simulink model "Trial_Merge_Unsuccessful"  (R2020b)
settings: Solver=VariableStepAuto  StartTime=0.0  StopTime=10.0  RelTol=1e-3
values from neighbouring files (symbols this model uses):
  A_2 = zeros(3)    [MPC_tune.m]
  B_2 = I_inv    [MPC_tune.m]
  C_2 = eye(3)    [MPC_tune.m]
  D_2 = zeros(3)    [MPC_tune.m]
  I_inv = inv(I_mat)    [MPC_tune.m]
undefined symbols (not defined in the file or in its folder): Fb1_l, Fb1_u, Fb2_l, Fb2_u, Fb3_l, Fb3_u, Fb4_l, Fb4_u, Fc1_l, Fc1_u, Fc2_l, Fc2_u, Fc3_l, Fc3_u, fprop, Ft1_l, Ft1_u, Ft2_l, Ft2_u, Ft3_l, Ft3_u, Ft4_l, Ft4_u, theta0
libraries: dspsigops x33, pid_lib x3, fuzblock x3, mpclib x1, dspmathops x1
(part 2 of 2)

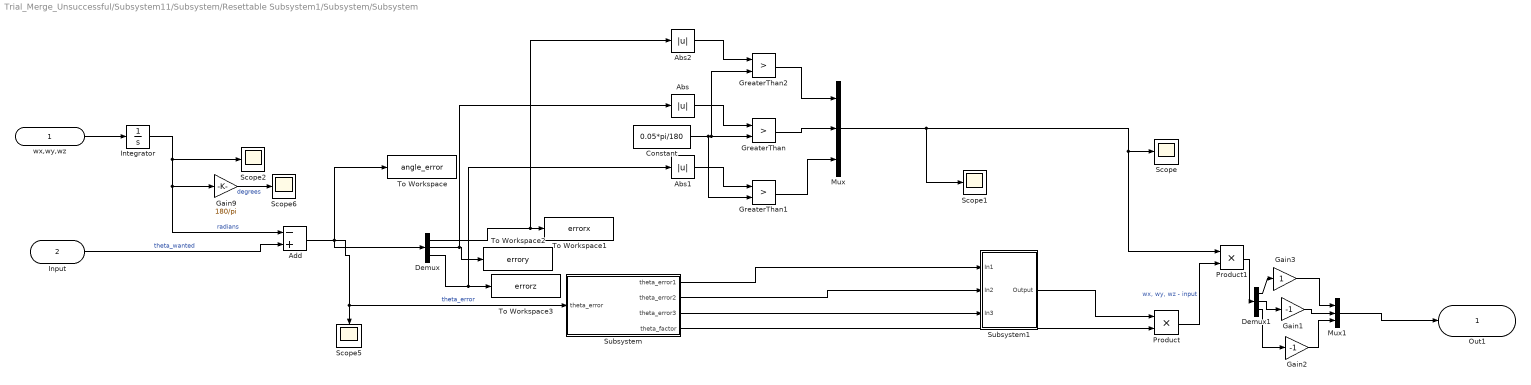
== system Trial_Merge_Unsuccessful/Subsystem11/Subsystem/Resettable Subsystem1/Subsystem/Subsystem ==
  wx,wy,wz : Inport
  Input : Inport  Port=2
  Abs : Abs
  Abs1 : Abs
  Abs2 : Abs
  Add : Sum  Inputs=-+
  Constant : Constant  Value=0.05*pi/180
  Demux : Demux  Outputs=3
  Demux1 : Demux  Outputs=3
  Gain1 : Gain  Gain=-1
  Gain2 : Gain  Gain=-1
  Gain3 : Gain
  Gain9 : Gain  Gain=180/pi
  GreaterThan : RelationalOperator  Operator=>  OutDataTypeStr=boolean  RndMeth=Simplest
  GreaterThan1 : RelationalOperator  Operator=>  OutDataTypeStr=boolean  RndMeth=Simplest
  GreaterThan2 : RelationalOperator  Operator=>  OutDataTypeStr=boolean  RndMeth=Simplest
  Integrator : Integrator  InitialCondition=[0;0;0]
  Mux : Mux  Inputs=3
  Mux1 : Mux  Inputs=3
  Product : Product
  Product1 : Product
  Scope{,1..2,5..6} (5 alike) : Scope
  Subsystem : Subsystem
  Subsystem1 : Subsystem
  To Workspace : ToWorkspace  VariableName=angle_error  SampleTime=-1
  To Workspace1 : ToWorkspace  VariableName=errorx  SaveFormat=Timeseries  SampleTime=-1
      settings: Save2DSignal=2-D array (concatenate along first dimension)
  To Workspace2 : ToWorkspace  VariableName=errory  SaveFormat=Timeseries  SampleTime=-1
  To Workspace3 : ToWorkspace  VariableName=errorz  SaveFormat=Timeseries  SampleTime=-1
  Out1 : Outport
  wires:
  Integrator/1 -> Add/1, Gain9/1, Scope2/1  "radians"
  Add/1 -> To Workspace/1, Demux/1, Subsystem/1(theta_error), Scope5/1  "theta_error"
  Gain9/1 -> Scope6/1  "degrees"
  Input/1 -> Add/2  "theta_wanted"
  Product/1 -> Product1/2  "wx, wy, wz - input"
  wx,wy,wz/1 -> Integrator/1
  Subsystem/4(theta_factor) -> Product/2
  Demux/2 -> Abs/1, To Workspace2/1
  Demux/3 -> Abs1/1, To Workspace3/1
  Demux/1 -> Abs2/1, To Workspace1/1
  Subsystem/1(theta_error1) -> Subsystem1/1(In1)
  Subsystem/2(theta_error2) -> Subsystem1/2(In2)
  Subsystem/3(theta_error3) -> Subsystem1/3(In3)
  Subsystem1/1(Output) -> Product/1
  Abs/1 -> GreaterThan/1
  Constant/1 -> GreaterThan1/2, GreaterThan2/2, GreaterThan/2
  Abs1/1 -> GreaterThan1/1
  Abs2/1 -> GreaterThan2/1
  GreaterThan2/1 -> Mux/1
  GreaterThan/1 -> Mux/2
  GreaterThan1/1 -> Mux/3
  Mux/1 -> Scope1/1, Scope/1, Product1/1
  Product1/1 -> Demux1/1
  Mux1/1 -> Out1/1
  Demux1/2 -> Gain1/1
  Demux1/3 -> Gain2/1
  Demux1/1 -> Gain3/1
  Gain3/1 -> Mux1/1
  Gain1/1 -> Mux1/2
  Gain2/1 -> Mux1/3

== system Trial_Merge_Unsuccessful/Subsystem11/Subsystem/Resettable Subsystem1/Subsystem/Subsystem1 ==
  u : Inport
  A : Inport  Port=2
  B : Inport  Port=3
  C : Inport  Port=4
  D : Inport  Port=5
  w_0 : Inport  Port=6
  Input : Inport  Port=7
  Product{,1..3} (4 alike) : Product  SCDEnableBlockLinearizationSpecification=on  Multiplication=Matrix(*)
  Resettable Subsystem : Subsystem  TreatAsAtomicUnit=on
  Sum : Sum  Inputs=|++
  Sum1 : Sum  Inputs=++|
  dxTerm : Terminator
  y : Outport  VectorParamsAs1DForOutWhenUnconnected=off
  x : Outport  Port=2  VectorParamsAs1DForOutWhenUnconnected=off
  wires:
  Sum/1 -> Resettable Subsystem/1(alpha), dxTerm/1  "dx"
  Product3/1 -> Sum1/1  "Cx"
  Product/1 -> Sum/1  "Bu"
  u/1 -> Product2/2, Product/2
  Product2/1 -> Sum1/2  "Du"
  Resettable Subsystem/1(x) -> x/1, Product1/2, Product3/2  "x"
  A/1 -> Product1/1
  Product1/1 -> Sum/2  "Ax"
  C/1 -> Product3/1
  B/1 -> Product/1
  D/1 -> Product2/1
  Sum1/1 -> y/1
  w_0/1 -> Resettable Subsystem/2(omega0)
  Input/1 -> Resettable Subsystem/Reset

== system Trial_Merge_Unsuccessful/Subsystem11/Subsystem/Resettable Subsystem1/Subsystem1/Subsystem ==
  F_c_d : Inport
  M_c_d : Inport  Port=2
  Demux8 : Demux  Outputs=3
  Demux9 : Demux  Outputs=3
  MATLAB Function : MATLAB Function  TreatAsAtomicUnit=on
  MATLAB Function6 : MATLAB Function  TreatAsAtomicUnit=on
  Mux23 : Mux
  Mux24 : Mux
  Mux9 : Mux  Inputs=3
  Terminator12 : Terminator
  To Workspace6 : ToWorkspace  VariableName=Fc_wanted  SaveFormat=Timeseries  SampleTime=-1
  To Workspace7 : ToWorkspace  VariableName=Ft_wanted  SaveFormat=Timeseries  SampleTime=-1
  To Workspace8 : ToWorkspace  VariableName=Fb_wanted  SaveFormat=Timeseries  SampleTime=-1
  Fb_wanted : Outport
  Ft_wanted : Outport  Port=2
  Fc_wanted : Outport  Port=3
  wires:
  Demux9/3 -> MATLAB Function6/3(M_z)
  Demux8/2 -> MATLAB Function6/1(F_y)
  Mux9/1 -> Fc_wanted/1, To Workspace6/1  "Fc_wanted"
  MATLAB Function/2(Ft2) -> Mux23/2  "Fb_wanted"
  Demux9/1 -> MATLAB Function6/2(M_x)
  MATLAB Function/3(Ft3) -> Mux23/3
  Demux9/2 -> MATLAB Function/1(My)
  MATLAB Function/8(Fb4) -> Mux24/4
  MATLAB Function6/1(F_c1) -> Mux9/1
  MATLAB Function/1(Ft1) -> Mux23/1  "Ft_wanted"
  Demux8/1 -> Terminator12/1
  Mux23/1 -> Ft_wanted/1, To Workspace7/1  "Ft_wanted"
  Mux24/1 -> Fb_wanted/1, To Workspace8/1  "Fb_wanted"
  MATLAB Function6/3(F_c3) -> Mux9/3
  MATLAB Function/5(Fb1) -> Mux24/1
  MATLAB Function/6(Fb2) -> Mux24/2
  MATLAB Function/7(Fb3) -> Mux24/3
  MATLAB Function/4(Ft4) -> Mux23/4
  Demux8/3 -> MATLAB Function/2(Fz)
  MATLAB Function6/2(F_c2) -> Mux9/2
  F_c_d/1 -> Demux8/1
  M_c_d/1 -> Demux9/1

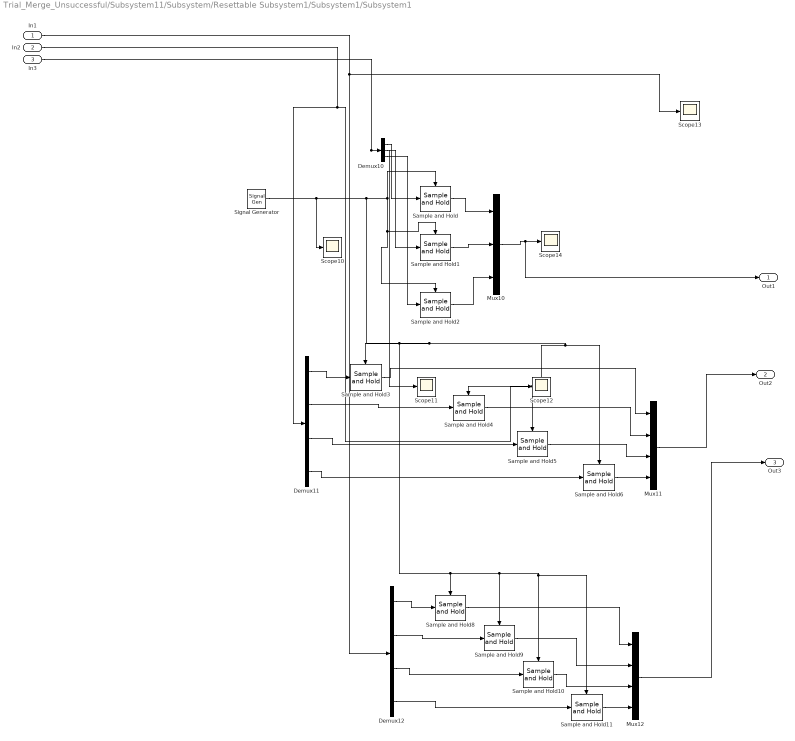
== system Trial_Merge_Unsuccessful/Subsystem11/Subsystem/Resettable Subsystem1/Subsystem1/Subsystem1 ==
  In1 : Inport
  In2 : Inport  Port=2
  In3 : Inport  Port=3
  Demux10 : Demux  Outputs=3
  Demux11 : Demux
  Demux12 : Demux
  Mux10 : Mux  Inputs=3
  Mux11 : Mux
  Mux12 : Mux
  Sample and Hold{,1..6,8..11} (11 alike) : dspsigops/Sample and Hold  trig=Rising edge  initCond=0  latchinput=off
  Scope{10..14} (5 alike) : Scope
  Signal Generator : SignalGenerator  WaveForm=square  Frequency=fprop  Units=rad/sec
  Out1 : Outport
  Out2 : Outport  Port=2
  Out3 : Outport  Port=3
  wires:
  Demux12/1 -> Sample and Hold8/1
  Demux11/1 -> Sample and Hold3/1
  Signal Generator/1 -> Scope10/1, Sample and Hold11/Trigger, Sample and Hold10/Trigger, Sample and Hold9/Trigger, Sample and Hold8/Trigger, Sample and Hold4/Trigger, Sample and Hold5/Trigger, Sample and Hold6/Trigger, Sample and Hold3/Trigger, Sample and Hold/Trigger, Sample and Hold2/Trigger, Sample and Hold1/Trigger
  In2/1 -> Scope12/1, Demux11/1
  In3/1 -> Scope11/1, Demux10/1
  Demux10/3 -> Sample and Hold2/1
  Sample and Hold10/1 -> Mux12/3
  Sample and Hold/1 -> Mux10/1
  Demux12/4 -> Sample and Hold11/1
  Sample and Hold6/1 -> Mux11/4
  Demux10/1 -> Sample and Hold/1
  Mux10/1 -> Out1/1, Scope14/1
  Demux12/3 -> Sample and Hold10/1
  Sample and Hold8/1 -> Mux12/1
  Sample and Hold3/1 -> Mux11/1
  Sample and Hold5/1 -> Mux11/3
  Sample and Hold1/1 -> Mux10/2
  Sample and Hold11/1 -> Mux12/4
  In1/1 -> Scope13/1, Demux12/1
  Demux10/2 -> Sample and Hold1/1
  Demux11/2 -> Sample and Hold4/1
  Sample and Hold2/1 -> Mux10/3
  Sample and Hold4/1 -> Mux11/2
  Sample and Hold9/1 -> Mux12/2
  Demux11/3 -> Sample and Hold5/1
  Mux12/1 -> Out3/1
  Demux12/2 -> Sample and Hold9/1
  Demux11/4 -> Sample and Hold6/1
  Mux11/1 -> Out2/1

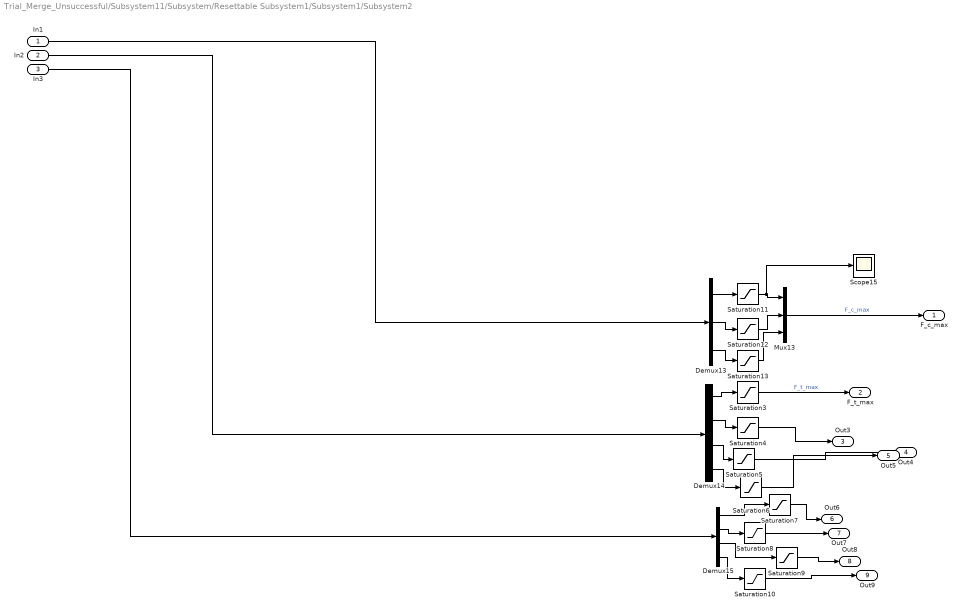
== system Trial_Merge_Unsuccessful/Subsystem11/Subsystem/Resettable Subsystem1/Subsystem1/Subsystem2 ==
  In1 : Inport
  In2 : Inport  Port=2
  In3 : Inport  Port=3
  Demux13 : Demux  Outputs=3
  Demux14 : Demux
  Demux15 : Demux
  Mux13 : Mux  Inputs=3
  Saturation10 : Saturate  UpperLimit=Fb4_u  LowerLimit=Fb4_l
  Saturation11 : Saturate  UpperLimit=Fc1_u  LowerLimit=Fc1_l
  Saturation12 : Saturate  UpperLimit=Fc2_u  LowerLimit=Fc2_l
  Saturation13 : Saturate  UpperLimit=Fc3_u  LowerLimit=Fc3_l
  Saturation3 : Saturate  UpperLimit=Ft1_u  LowerLimit=Ft1_l
  Saturation4 : Saturate  UpperLimit=Ft2_u  LowerLimit=Ft2_l
  Saturation5 : Saturate  UpperLimit=Ft3_u  LowerLimit=Ft3_l
  Saturation6 : Saturate  UpperLimit=Ft4_u  LowerLimit=Ft4_l
  Saturation7 : Saturate  UpperLimit=Fb1_u  LowerLimit=Fb1_l
  Saturation8 : Saturate  UpperLimit=Fb2_u  LowerLimit=Fb2_l
  Saturation9 : Saturate  UpperLimit=Fb3_u  LowerLimit=Fb3_l
  Scope15 : Scope
  F_c_max : Outport
  F_t_max : Outport  Port=2
  Out3 : Outport  Port=3
  Out4 : Outport  Port=4
  Out5 : Outport  Port=5
  Out6 : Outport  Port=6
  Out7 : Outport  Port=7
  Out8 : Outport  Port=8
  Out9 : Outport  Port=9
  wires:
  Saturation11/1 -> Scope15/1, Mux13/1
  Demux13/2 -> Saturation12/1
  Saturation10/1 -> Out9/1
  Demux13/3 -> Saturation13/1
  Demux14/1 -> Saturation3/1
  Demux14/4 -> Saturation6/1
  In3/1 -> Demux15/1
  Demux14/3 -> Saturation5/1
  Demux13/1 -> Saturation11/1
  Saturation13/1 -> Mux13/3
  In1/1 -> Demux13/1
  Demux15/1 -> Saturation7/1
  Demux15/2 -> Saturation8/1
  Demux15/3 -> Saturation9/1
  Saturation12/1 -> Mux13/2
  Demux15/4 -> Saturation10/1
  Demux14/2 -> Saturation4/1
  Saturation9/1 -> Out8/1
  Saturation5/1 -> Out4/1
  In2/1 -> Demux14/1
  Saturation4/1 -> Out3/1
  Saturation7/1 -> Out6/1
  Mux13/1 -> F_c_max/1  "F_c_max"
  Saturation6/1 -> Out5/1
  Saturation3/1 -> F_t_max/1  "F_t_max"
  Saturation8/1 -> Out7/1

== system Trial_Merge_Unsuccessful/Subsystem11/Subsystem/Resettable Subsystem1/Subsystem1/Subsystem3 ==
  In1 : Inport
  In2 : Inport  Port=2
  In3 : Inport  Port=3
  Ft3 : Inport  Port=4
  Ft4 : Inport  Port=5
  Fb1 : Inport  Port=6
  In7 : Inport  Port=7
  Fb3 : Inport  Port=8
  In9 : Inport  Port=9
  Constant23 : Constant  Value=0
  Demux16 : Demux  Outputs=3
  MATLAB Function7 : MATLAB Function  TreatAsAtomicUnit=on
  MATLAB Function8 : MATLAB Function  TreatAsAtomicUnit=on
  MATLAB Function9 : MATLAB Function  TreatAsAtomicUnit=on
  Mux : Mux
  Mux1 : Mux
  Mux16 : Mux  Inputs=3
  Mux17 : Mux  Inputs=3
  To Workspace : ToWorkspace  VariableName=Fc  SaveFormat=Timeseries  SampleTime=-1
  To Workspace1 : ToWorkspace  VariableName=Ft  SaveFormat=Timeseries  SampleTime=-1
  To Workspace2 : ToWorkspace  VariableName=Fb  SaveFormat=Timeseries  SampleTime=-1
  Out1 : Outport
  Mc(t-tau)_actual : Outport  Port=2
  wires:
  Demux16/2 -> MATLAB Function8/2(F_c2)
  In9/1 -> Mux1/4, MATLAB Function9/8(Fb4)
  In3/1 -> Mux/2, MATLAB Function9/2(Ft2)
  MATLAB Function7/1(F_z) -> Mux16/3  "Fz_actual"
  In1/1 -> Demux16/1, To Workspace/1
  Fb3/1 -> Mux1/3, MATLAB Function9/7(Fb3)
  MATLAB Function9/1(F1) -> MATLAB Function7/1(F1)
  Ft3/1 -> Mux/3, MATLAB Function9/3(Ft3)
  MATLAB Function8/1(F_y) -> Mux16/2  "Fy_actual"
  Fb1/1 -> Mux1/1, MATLAB Function9/5(Fb1)
  MATLAB Function8/3(M_z) -> Mux17/3  "M_z_acc"
  MATLAB Function7/2(M_y) -> Mux17/2  "M_y_acc"
  Mux17/1 -> Mc(t-tau)_actual/1  "Mc(t-tau)_actual"
  Ft4/1 -> Mux/4, MATLAB Function9/4(Ft4)
  MATLAB Function8/2(M_x) -> Mux17/1  "M_x_acc"
  In7/1 -> Mux1/2, MATLAB Function9/6(Fb2)
  MATLAB Function9/3(F3) -> MATLAB Function7/3(F3)
  Demux16/1 -> MATLAB Function8/1(F_c1)
  Constant23/1 -> Mux16/1  "Fx_actual"
  In2/1 -> Mux/1, MATLAB Function9/1(Ft1)
  MATLAB Function9/2(F2) -> MATLAB Function7/2(F2)
  Mux1/1 -> To Workspace2/1
  Demux16/3 -> MATLAB Function8/3(F_c3)
  Mux/1 -> To Workspace1/1
  Mux16/1 -> Out1/1

== system Trial_Merge_Unsuccessful/Subsystem11/Subsystem/Resettable Subsystem1/Subsystem1/Subsystem4 ==
  TVd : Inport
  In2 : Inport  Port=2
  Constant24 : Constant  Value=[0;1;1]
  Matrix Multiply3 : Product  Multiplication=Matrix(*)
  Product5 : Product
  Fc(t-tau)_actual : Outport
  Fc(t-tau)_actual1 : Outport  Port=2
  wires:
  Matrix Multiply3/1 -> Fc(t-tau)_actual1/1, Product5/2  "Fc(t-tau)_actual"
  Constant24/1 -> Product5/1
  TVd/1 -> Matrix Multiply3/1
  Product5/1 -> Fc(t-tau)_actual/1  "Fc(t-tau)_actual"
  In2/1 -> Matrix Multiply3/2

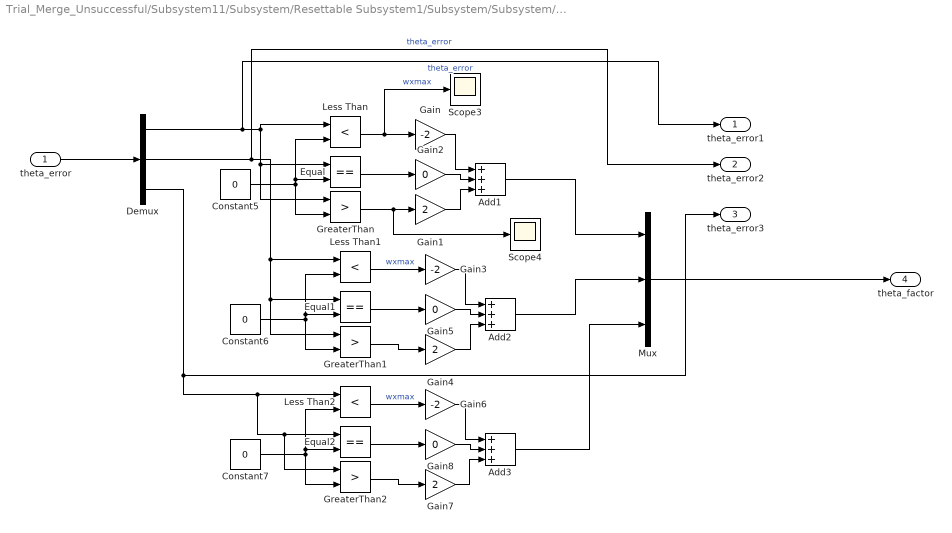
== system Trial_Merge_Unsuccessful/Subsystem11/Subsystem/Resettable Subsystem1/Subsystem/Subsystem/Subsystem ==
  theta_error : Inport
  Add1 : Sum  Inputs=+++
  Add2 : Sum  Inputs=+++
  Add3 : Sum  Inputs=+++
  Constant5 : Constant  Value=0
  Constant6 : Constant  Value=0
  Constant7 : Constant  Value=0
  Demux : Demux  Outputs=3
  Equal : RelationalOperator  Operator===  OutDataTypeStr=boolean  RndMeth=Simplest
  Equal1 : RelationalOperator  Operator===  OutDataTypeStr=boolean  RndMeth=Simplest
  Equal2 : RelationalOperator  Operator===  OutDataTypeStr=boolean  RndMeth=Simplest
  Gain : Gain  Gain=-2
  Gain1 : Gain  Gain=2
  Gain2 : Gain  Gain=0
  Gain3 : Gain  Gain=-2
  Gain4 : Gain  Gain=2
  Gain5 : Gain  Gain=0
  Gain6 : Gain  Gain=-2
  Gain7 : Gain  Gain=2
  Gain8 : Gain  Gain=0
  GreaterThan : RelationalOperator  Operator=>  OutDataTypeStr=boolean  RndMeth=Simplest
  GreaterThan1 : RelationalOperator  Operator=>  OutDataTypeStr=boolean  RndMeth=Simplest
  GreaterThan2 : RelationalOperator  Operator=>  OutDataTypeStr=boolean  RndMeth=Simplest
  Less Than : RelationalOperator  Operator=<  OutDataTypeStr=boolean  RndMeth=Simplest
  Less Than1 : RelationalOperator  Operator=<  OutDataTypeStr=boolean  RndMeth=Simplest
  Less Than2 : RelationalOperator  Operator=<  OutDataTypeStr=boolean  RndMeth=Simplest
  Mux : Mux  Inputs=3
  Scope3 : Scope
  Scope4 : Scope
  theta_error1 : Outport
  theta_error2 : Outport  Port=2
  theta_error3 : Outport  Port=3
  theta_factor : Outport  Port=4
  wires:
  Add1/1 -> Mux/1
  Constant5/1 -> Equal/2, Less Than/2, GreaterThan/2
  Equal2/1 -> Gain8/1
  Demux/1 -> theta_error1/1, GreaterThan/1, Equal/1, Less Than/1  "theta_error"
  GreaterThan2/1 -> Gain7/1
  Gain1/1 -> Add1/3
  Gain7/1 -> Add3/3
  Less Than1/1 -> Gain3/1  "wxmax"
  Gain6/1 -> Add3/1
  Equal/1 -> Gain2/1
  Gain5/1 -> Add2/2
  Add3/1 -> Mux/3
  GreaterThan/1 -> Scope4/1, Gain1/1
  Constant6/1 -> Equal1/2, Less Than1/2, GreaterThan1/2
  Demux/3 -> theta_error3/1, GreaterThan2/1, Equal2/1, Less Than2/1
  Gain3/1 -> Add2/1
  Constant7/1 -> Equal2/2, Less Than2/2, GreaterThan2/2
  Equal1/1 -> Gain5/1
  Gain8/1 -> Add3/2
  Gain4/1 -> Add2/3
  GreaterThan1/1 -> Gain4/1
  Gain/1 -> Add1/1
  Demux/2 -> theta_error2/1, GreaterThan1/1, Equal1/1, Less Than1/1  "theta_error"
  Gain2/1 -> Add1/2
  Add2/1 -> Mux/2
  Less Than/1 -> Scope3/1, Gain/1  "wxmax"
  Less Than2/1 -> Gain6/1  "wxmax"
  theta_error/1 -> Demux/1
  Mux/1 -> theta_factor/1

== system Trial_Merge_Unsuccessful/Subsystem11/Subsystem/Resettable Subsystem1/Subsystem/Subsystem/Subsystem1 ==
  In1 : Inport
  In2 : Inport  Port=2
  In3 : Inport  Port=3
  Abs : Abs
  Abs1 : Abs
  Abs2 : Abs
  Demux : Demux  Outputs=3
  Gain : Gain  Gain=10
  Gain1 : Gain  Gain=125
  Gain10 : Gain  Gain=125
  Gain2 : Gain  Gain=125
  Gain3 : Gain  Gain=10
  Gain4 : Gain  Gain=10
  Mux : Mux  Inputs=3
  Mux1 : Mux  Inputs=3
  Normalization : dspmathops/Normalization  NormType=Squared 2-norm  Bias=1e-10  NormOver=Each column  Dimension=1  roundingMode=Floor  overflowMode=off  accumDataTypeStr=Inherit: Same as product output  accumLastDataTypeStr=Inherit: Same as product output  outputDataTypeStr=Inherit: Same as product output  outputMin=[]  outputMax=[]  outputLastDataTypeStr=Inherit: Same as product output
  Scope{,1..7} (8 alike) : Scope
  Sigmoidal MF : fuzblock/Membership  Functions/Sigmoidal MF  a=10^(-8)  c=1000
      settings: SourceProductBaseCode=FL
  Sigmoidal MF1 : fuzblock/Membership  Functions/Sigmoidal MF  a=10^(-8)  c=1000
      settings: SourceProductBaseCode=FL
  Sigmoidal MF2 : fuzblock/Membership  Functions/Sigmoidal MF  a=10^(-8)  c=1000
      settings: SourceProductBaseCode=FL
  Output : Outport
  wires:
  Gain2/1 -> Mux/2
  Gain10/1 -> Mux/1
  Sigmoidal MF1/1 -> Gain1/1, Scope1/1
  Sigmoidal MF/1 -> Gain10/1, Scope7/1
  Sigmoidal MF2/1 -> Gain2/1, Scope3/1
  Gain/1 -> Scope/1, Sigmoidal MF/1
  Gain1/1 -> Mux/3
  Gain3/1 -> Scope2/1, Sigmoidal MF2/1
  In2/1 -> Abs1/1
  In1/1 -> Abs/1
  In3/1 -> Abs2/1
  Mux/1 -> Output/1
  Abs/1 -> Mux1/1
  Abs1/1 -> Mux1/2
  Gain4/1 -> Scope4/1, Sigmoidal MF1/1
  Abs2/1 -> Mux1/3
  Demux/3 -> Gain4/1
  Demux/1 -> Gain/1
  Demux/2 -> Gain3/1
  Mux1/1 -> Normalization/1, Scope6/1
  Normalization/1 -> Scope5/1, Demux/1

== system Trial_Merge_Unsuccessful/Subsystem11/Subsystem/Resettable Subsystem1/Subsystem/Subsystem1/Resettable Subsystem ==
  alpha : Inport
  omega0 : Inport  Port=2
  Reset : ResetPort  DisableCoverage=on
  Integrator : Integrator  InitialConditionSource=external  InitialCondition=theta0
  Scope : Scope
  x : Outport
  wires:
  omega0/1 -> Integrator/2
  alpha/1 -> Integrator/1
  Integrator/1 -> Scope/1, x/1

== matlab function Trial_Merge_Unsuccessful/Subsystem11/Subsystem/Resettable Subsystem/Subsystem/Subsystem3/MATLAB Function9 ==
  data: Ft1 input; F1 output; Ft2 input; F2 output; F3 output; Ft3 input; Ft4 input; Fb1 input; Fb2 input; Fb3 input; Fb4 input
function [F1, F2, F3] = fcn(Ft1, Ft2, Ft3, Ft4, Fb1, Fb2, Fb3, Fb4)
%F3 is one prop
%F1 is two props
%F2 is two props
F1 = 2*Ft1;
F2 = 2*Fb1;
F3 = Ft3;
end

== matlab function Trial_Merge_Unsuccessful/Subsystem5/MATLAB Function5 ==
  data: M_y input; F1 output; F_z input; F2 output; F3 output
function [F1, F2, F3] = fcn(M_y, F_z)
xt_1 = 1.2598;
xb_1 = 2.2598;
xt_3 = -1.3402;
x_t1 = xt_1;
x_b1 = xb_1;
x_t3 = xt_3;



A_mat = [1 1;
    xt_1 xb_1];

A_inv = inv(A_mat);

p_0 = 0.2;
p_minus1 = 0;
step = 1000;
Converged = 0;
p_list = [];
x_list = [];
y_list = [];
J_list = [];
Fzz =[];
Myy =[];
while Converged == 0
    B = [(F_z - 4*p_0); (M_y - 4*p_0*xt_3)];
    force_0 = (A_inv*B);
    J_0 = sqrt(force_0(1)^2 + force_0(2)^2 + p_0^2);
    back = A_mat*force_0;
    backtrack = [4*p_0; 4*p_0*xt_3];
    forceback = back+backtrack;
    diff = sum(abs(forceback - [F_z; M_y]));
    if diff > 10^(-7)
        disp('Error')
        break
    end
    force = force_0;
    J = J_0;
    p = p_0;
    
    p_1 = p_0 + step;
    B = [(F_z - 4*p_1); (M_y - 4*p_1*xt_3)];
    force_1 = (A_inv*B);
    J_1 = sqrt(force_1(1)^2 + force_1(2)^2 + p_1^2);
    back = A_mat*force_1;
    backtrack = [4*p_1; 4*p_1*xt_3];
    forceback = back+backtrack;
    diff = sum(abs(forceback - [F_z; M_y]));
    if diff > 10^(-7)
        disp('Error')
        break
    end
    if J_1 < J_0
        force = force_1;
        J = J_1;
        p = p_1;
    end
    
    p_2 = p_0 - step;
    B = [(F_z - 4*p_2); (M_y - 4*p_2*xt_3)];
    force_2 = (A_inv*B);
    J_2 = sqrt(force_2(1)^2 + force_2(2)^2 + p_2^2);
    back = A_mat*force_2;
    backtrack = [4*p_2; 4*p_2*xt_3];
    forceback = back+backtrack;
    diff = sum(abs(forceback - [F_z; M_y]));
    if diff > 10^(-7)
        disp('Error')
        break
    end
    if J_2 < J_0 && J_2 < J_1
        force = force_2;
        J = J_2;
        p = p_2;
    end
    
    if p_minus1 < p_0 && p_0 < p
        step = step;
    elseif p_minus1 > p_0 && p_0 > p
        step = step;
    else
        step = step*0.9;
    end
        
    p_minus1 = p_0;
    p_0 = p;
    p_list = [p_list; p_0];
    x_list = [x_list; force(1)];
    y_list = [y_list; force(2)];
    J_list = [J_list; J];
    if step < abs(min([F_z,M_y])*10^(-9))
        Converged = 1;
    end
    
    
end

F1 = x_list(length(x_list));
F2 = y_list(length(y_list));
F3 = p_0;
end

== matlab function Trial_Merge_Unsuccessful/Subsystem5/Subsystem/MATLAB Function6 ==
  data: F_y input; F_c1 output; M_x input; M_z input; F_c2 output; F_c3 output
function [F_c1, F_c2, F_c3] = fcn(F_y, M_x, M_z)
%CATIA trans
TcgCatia = [1 0 0;
    0 -1 0;
    0 0 -1];

%Propeller arms - changed due to CATIA errors
c_1 = [-640.1998; 0; 506.566]*10^(-3);      %Control Back Top
c_2 = [-1040.1998; 0; -493.434]*10^(-3);    %Control Back Bottom
c_3 = [2259.8002; 0; -293.434]*10^(-3);     %Control Front

%Propeller arms - rotated
c_1 = TcgCatia*c_1;
c1 = transpose(c_1);
c_2 = TcgCatia*c_2;
c2 = transpose(c_2);
c_3 = TcgCatia*c_3;
c3 = transpose(c_3);

xc_1 = c1(1);
zc_1 = c1(3);

xc_2 = c2(1);
zc_2 = c2(3);

xc_3 = c3(1);
zc_3 = c3(3);

A_control = [1 1 1;
    zc_1 zc_2 zc_3;
    xc_1 xc_2 xc_3];
A_cinv = inv(A_control);
force_control = [F_y; M_x; M_z];
controlvec = A_cinv*force_control;
F_c1 = controlvec(1);
F_c2 = controlvec(2);
F_c3 = controlvec(3);
end

== matlab function Trial_Merge_Unsuccessful/Subsystem5/MATLAB Function4 ==
  data: F1 input; F_t1 output; F2 input; F3 input; F_t2 output; F_t3 output; F_t4 output; F_b1 output; F_b2 output; F_b3 output; F_b4 output
function [F_t1, F_t2, F_t3, F_t4, F_b1, F_b2, F_b3, F_b4] = fcn(F1, F2, F3)
%F3 is one prop
%F1 is two props
%F2 is two props
F_t1 = F1/2;
F_t2 = F_t1;
F_t3 = F3;
F_t4 = F_t3;
F_b3 = F_t3;
F_b4 = F_t3;
F_b1 = F2/2;
F_b2 = F_b1;

Ft = [F_t1, F_t2, F_t3, F_t4];
Fb = [F_b1, F_b2, F_b3, F_b4];
end

== matlab function Trial_Merge_Unsuccessful/Subsystem5/Subsystem3/MATLAB Function7 ==
  data: F1 input; F_z output; F2 input; M_y output; F3 input
function [F_z, M_y] = fcn(F1, F2, F3)
xt_1 = 1.2598;
xb_1 = 2.2598;
xt_3 = -1.3402;
x_t1 = xt_1;
x_b1 = xb_1;
x_t3 = xt_3;

M_y = -100;
F_z = 0;

A_mat = [1 1;
    xt_1 xb_1];

A_inv = inv(A_mat);

force = [F1; F2];

back = A_mat*force;
backtrack = [4*F3; 4*F3*xt_3];
forceback = back+backtrack;
F_z = forceback(1);
M_y = forceback(2) + 0.15;
end

== matlab function Trial_Merge_Unsuccessful/Subsystem5/Subsystem3/MATLAB Function8 ==
  data: F_c1 input; F_y output; M_x output; F_c2 input; F_c3 input; M_z output
function [F_y, M_x, M_z] = fcn(F_c1, F_c2, F_c3)

%CATIA trans
TcgCatia = [1 0 0;
    0 -1 0;
    0 0 -1];

%Propeller arms - changed due to CATIA errors
c_1 = [-640.1998; 0; 506.566]*10^(-3);      %Control Back Top
c_2 = [-1040.1998; 0; -493.434]*10^(-3);    %Control Back Bottom
c_3 = [2259.8002; 0; -293.434]*10^(-3);     %Control Front

%Propeller arms - rotated
c_1 = TcgCatia*c_1;
c1 = transpose(c_1);
c_2 = TcgCatia*c_2;
c2 = transpose(c_2);
c_3 = TcgCatia*c_3;
c3 = transpose(c_3);

xc_1 = c1(1);
zc_1 = c1(3);

xc_2 = c2(1);
zc_2 = c2(3);

xc_3 = c3(1);
zc_3 = c3(3);


Control_forces = [F_c1; F_c2; F_c3];

A_control = [1 1 1;
        zc_1 zc_2 zc_3;
        xc_1 xc_2 xc_3]; 
Control_vec_2 = A_control*Control_forces;
F_y = Control_vec_2(1);
M_x = Control_vec_2(2);
M_z = Control_vec_2(3);
end

== matlab function Trial_Merge_Unsuccessful/Subsystem5/Subsystem3/MATLAB Function9 ==
  data: Ft1 input; F1 output; Ft2 input; F2 output; F3 output; Ft3 input; Ft4 input; Fb1 input; Fb2 input; Fb3 input; Fb4 input
function [F1, F2, F3] = fcn(Ft1, Ft2, Ft3, Ft4, Fb1, Fb2, Fb3, Fb4)
%F3 is one prop
%F1 is two props
%F2 is two props
F1 = 2*Ft1;
F2 = 2*Fb1;
F3 = Ft3;
end

== matlab function Trial_Merge_Unsuccessful/Subsystem11/Subsystem/Resettable Subsystem/Subsystem/MATLAB Function4 ==
  data: F1 input; F_t1 output; F2 input; F3 input; F_t2 output; F_t3 output; F_t4 output; F_b1 output; F_b2 output; F_b3 output; F_b4 output
function [F_t1, F_t2, F_t3, F_t4, F_b1, F_b2, F_b3, F_b4] = fcn(F1, F2, F3)
%F3 is one prop
%F1 is two props
%F2 is two props
F_t1 = F1/2;
F_t2 = F_t1;
F_t3 = F3;
F_t4 = F_t3;
F_b3 = F_t3;
F_b4 = F_t3;
F_b1 = F2/2;
F_b2 = F_b1;

Ft = [F_t1, F_t2, F_t3, F_t4];
Fb = [F_b1, F_b2, F_b3, F_b4];
end

== matlab function Trial_Merge_Unsuccessful/Subsystem11/Subsystem/Resettable Subsystem/Subsystem4/MATLAB Function2 ==
  data: theta_x input; Transformation_Mat output; theta_y input; theta_z input
function Transformation_Mat  = Euler(theta_x, theta_y, theta_z)

a = cos(theta_x)*cos(theta_z);
b = cos(theta_x)*sin(theta_z);
c = - sin(theta_x);
d = sin(theta_y)*sin(theta_x)*cos(theta_z) - cos(theta_y)*sin(theta_z);
e = sin(theta_y)*sin(theta_x)*sin(theta_z) + cos(theta_y)*cos(theta_z);
f = sin(theta_y)*cos(theta_x);
g = cos(theta_y)*sin(theta_x)*cos(theta_z) + sin(theta_y)*sin(theta_z);
h = cos(theta_y)*sin(theta_x)*sin(theta_z) - sin(theta_y)*cos(theta_z);
i = cos(theta_y)*cos(theta_x);

Transformation_Mat = [a b c;
    d e f;
    g h i];


end

== matlab function Trial_Merge_Unsuccessful/Subsystem11/Subsystem/Resettable Subsystem/Subsystem4/MATLAB Function3 ==
  data: theta_x input; Transformation_Mat output; theta_y input; theta_z input
function Transformation_Mat  = Euler(theta_x, theta_y, theta_z)

a = cos(theta_x)*cos(theta_z);
b = cos(theta_x)*sin(theta_z);
c = - sin(theta_x);
d = sin(theta_y)*sin(theta_x)*cos(theta_z) - cos(theta_y)*sin(theta_z);
e = sin(theta_y)*sin(theta_x)*sin(theta_z) + cos(theta_y)*cos(theta_z);
f = sin(theta_y)*cos(theta_x);
g = cos(theta_y)*sin(theta_x)*cos(theta_z) + sin(theta_y)*sin(theta_z);
h = cos(theta_y)*sin(theta_x)*sin(theta_z) - sin(theta_y)*cos(theta_z);
i = cos(theta_y)*cos(theta_x);

Transformation_Mat = [a b c;
    d e f;
    g h i];


end

== matlab function Trial_Merge_Unsuccessful/Subsystem11/Subsystem/Resettable Subsystem/Subsystem3/MATLAB Function10 ==
  settings: updateMethod=DISCRETE
  data: xvel input; yvel input; zvel input; wx output; accx input; accy input; accz input; wy output; wz output
function [wx, wy, wz]  = fungyroscope(xvel, yvel, zvel, accx, accy, accz)
   
    % Create gyroscope sensor object
    params = gyroparams;         
    
    % Parameters for simulated signal
    N = 1;       % Number of samples
    Fs = 100;       % Sampling rate
    Fc = 0.25;      % Sinusoidal frequency
    
    % Create arrays
    t = (0:(1/Fs):((N-1)/Fs)).';
    acc = [accx, accy, accz];          % Input accelerations
    angvel = [xvel,yvel,zvel];
    %angvel(:,1) = 8*sin(2*pi*Fc*t);
    
    % Generate gyroscopic data
    imu = imuSensor('SampleRate', Fs, 'Gyroscope', params);
    %imu.Gyroscope.MeasurementRange = 1000;   % Maximum angular velocity gyroscope can measure
    %imu.Gyroscope.Resolution = 1/Fs;           % Step size of digital measurements
    
    % Biases
    
    %imu.Gyroscope.BiasInstability = 0.012 * 3.14159 / 180;       % rad/hr
    %imu.Gyroscope.NoiseDensity = 0.15 * 3.14159 / 180;          % rad/s
    %imu.Gyroscope.RandomWalk = 0.017 * 3.14159 / 180;           % rad/sqrt(hr)
    %imu.Gyroscope.TemperatureBias = 0.25 * 3.14159 / 180;       % rad/s
    %imu.Gyroscope.AccelerationBias = 0.3;
    
    % Define real accelerations
    %acc(:,1) = 1;
    [~, gyroData] = imu(acc, angvel, eye(3));
    
    wx = gyroData(1);
    wy = gyroData(2);
    wz = gyroData(3);

end

== matlab function Trial_Merge_Unsuccessful/Subsystem11/Subsystem/Resettable Subsystem1/Subsystem1/MATLAB Function4 ==
  data: F1 input; F_t1 output; F2 input; F3 input; F_t2 output; F_t3 output; F_t4 output; F_b1 output; F_b2 output; F_b3 output; F_b4 output
function [F_t1, F_t2, F_t3, F_t4, F_b1, F_b2, F_b3, F_b4] = fcn(F1, F2, F3)
%F3 is one prop
%F1 is two props
%F2 is two props
F_t1 = F1/2;
F_t2 = F_t1;
F_t3 = F3;
F_t4 = F_t3;
F_b3 = F_t3;
F_b4 = F_t3;
F_b1 = F2/2;
F_b2 = F_b1;

Ft = [F_t1, F_t2, F_t3, F_t4];
Fb = [F_b1, F_b2, F_b3, F_b4];
end

== matlab function Trial_Merge_Unsuccessful/Subsystem11/Subsystem/Resettable Subsystem1/Subsystem1/MATLAB Function5 ==
  data: M_y input; F1 output; F_z input; F2 output; F3 output
function [F1, F2, F3] = fcn(M_y, F_z)
xt_1 = 1.2598;
xb_1 = 2.2598;
xt_3 = -1.3402;
x_t1 = xt_1;
x_b1 = xb_1;
x_t3 = xt_3;



A_mat = [1 1;
    xt_1 xb_1];

A_inv = inv(A_mat);

p_0 = 0.2;
p_minus1 = 0;
step = 1000;
Converged = 0;
p_list = [];
x_list = [];
y_list = [];
J_list = [];
Fzz =[];
Myy =[];
while Converged == 0
    B = [(F_z - 4*p_0); (M_y - 4*p_0*xt_3)];
    force_0 = (A_inv*B);
    J_0 = sqrt(force_0(1)^2 + force_0(2)^2 + p_0^2);
    back = A_mat*force_0;
    backtrack = [4*p_0; 4*p_0*xt_3];
    forceback = back+backtrack;
    diff = sum(abs(forceback - [F_z; M_y]));
    if diff > 10^(-7)
        disp('Error')
        break
    end
    force = force_0;
    J = J_0;
    p = p_0;
    
    p_1 = p_0 + step;
    B = [(F_z - 4*p_1); (M_y - 4*p_1*xt_3)];
    force_1 = (A_inv*B);
    J_1 = sqrt(force_1(1)^2 + force_1(2)^2 + p_1^2);
    back = A_mat*force_1;
    backtrack = [4*p_1; 4*p_1*xt_3];
    forceback = back+backtrack;
    diff = sum(abs(forceback - [F_z; M_y]));
    if diff > 10^(-7)
        disp('Error')
        break
    end
    if J_1 < J_0
        force = force_1;
        J = J_1;
        p = p_1;
    end
    
    p_2 = p_0 - step;
    B = [(F_z - 4*p_2); (M_y - 4*p_2*xt_3)];
    force_2 = (A_inv*B);
    J_2 = sqrt(force_2(1)^2 + force_2(2)^2 + p_2^2);
    back = A_mat*force_2;
    backtrack = [4*p_2; 4*p_2*xt_3];
    forceback = back+backtrack;
    diff = sum(abs(forceback - [F_z; M_y]));
    if diff > 10^(-7)
        disp('Error')
        break
    end
    if J_2 < J_0 && J_2 < J_1
        force = force_2;
        J = J_2;
        p = p_2;
    end
    
    if p_minus1 < p_0 && p_0 < p
        step = step;
    elseif p_minus1 > p_0 && p_0 > p
        step = step;
    else
        step = step*0.9;
    end
        
    p_minus1 = p_0;
    p_0 = p;
    p_list = [p_list; p_0];
    x_list = [x_list; force(1)];
    y_list = [y_list; force(2)];
    J_list = [J_list; J];
    if step < abs(min([F_z,M_y])*10^(-9))
        Converged = 1;
    end
    
    
end

F1 = x_list(length(x_list));
F2 = y_list(length(y_list));
F3 = p_0;
end

== matlab function Trial_Merge_Unsuccessful/Subsystem11/Subsystem/Resettable Subsystem1/Subsystem1/Subsystem/MATLAB Function ==
  data: My input; Ft1 output; Fz input; Ft2 output; Ft3 output; Ft4 output; Fb1 output; Fb2 output; Fb3 output; Fb4 output
function [Ft1, Ft2, Ft3, Ft4, Fb1, Fb2, Fb3, Fb4] = fixingpropulsionsmess(My, Fz)
xt_1 = 1.2598;
xb_1 = 2.2598;
xt_3 = -1.3402;
xb_3 = -1.3402;
x_t1 = xt_1;
x_b1 = xb_1;
x_t3 = xt_3;
x_b3 = xb_3;;

%alpha_1 = (-2*xt_1*(1/((xt_1/xb_1)-1))*(2 - (2*xb_3/xb_1)) - 4*xb_3)^2;
%alpha_2 = ((1/((xt_1/xb_1)-1))*(2-(2*xb_3/xb_1)))^2;
%alpha = alpha_1 + alpha_2;

%beta_1 = 2*My*((1/(2*xb_1))*(1 - (xt_1/xb_1)*(1/((xt_1/xb_1) -1))));
%beta_2 = 2*My*(1/((xt_1/xb_1) -1))*(1/(2*xb_1))*(1/((xt_1/xb_1) -1))*(2 - ((2*xb_3)/x_b1));
%beta_3 = 2*Fz*(1/(2*xb_1)*xt_1*(1/(xt_1/xb_1 -1)));
%beta_4 = 2*Fz*(-1/2*(1/(xt_1/xb_1 -1))*(1/(xt_1/xb_1 -1))*(2-2*xb_3/xb_1));
%beta = beta_1 + beta_2 + beta_3 + beta_4;

%a = beta/(2*alpha);
%y = 1/(2*xb_1)*(My - 2*xt_1*(1/(xt_1/xb_1 -1))*(-0.5*Fz + 2*(2 - 2*xb_3/xb_1)*a + 1/(2*xb_1)*My) - 4*xb_3*a);
%x = (1/(xt_1/xb_1 -1))*(-0.5*Fz + (2 - 2*xb_3/xb_1)*a + 1/(2*xb_1)*My);

a_num = 2/((2*xb_1 - 2*xt_1)^2) *(2*(4*xt_1 - 4*xb_3)*(My - Fz*0.5)) + 2*Fz + (4*My - Fz*(2 + 4*xt_1 - 4*xb_3))/(2*xb_1 - 2*xt_1);
a_den = -(2/((2*xb_1 - 2*xt_1)^2)*2*((4*xt_1 - 4*xb_3)^2) + 10 + (8*(4*xt_1 - 4*xb_3))/(-2*xt_1 + 2*xb_1));
a = a_num/a_den;

y = 1/(-2*xt_1 + 2*xb_1)*(a*(4*xt_1 - 4*xb_3) + My - 0.5*Fz);
x = -y - 2*a + Fz/2;
z = a;

Ft1 = x;
Ft2 = Ft1;
Ft3 = a;
Ft4 = Ft3;
Fb1 = y;
Fb2 = Fb1;
Fb3 = Ft3;
Fb4 = Ft3;
end

== matlab function Trial_Merge_Unsuccessful/Subsystem11/Subsystem/Resettable Subsystem1/Subsystem1/Subsystem/MATLAB Function6 ==
  data: F_y input; F_c1 output; M_x input; M_z input; F_c2 output; F_c3 output
function [F_c1, F_c2, F_c3] = fcn(F_y, M_x, M_z)
%CATIA trans
TcgCatia = [1 0 0;
    0 -1 0;
    0 0 -1];

%Propeller arms - changed due to CATIA errors
c_1 = [-640.1998; 0; 506.566]*10^(-3);      %Control Back Top
c_2 = [-1040.1998; 0; -493.434]*10^(-3);    %Control Back Bottom
c_3 = [2259.8002; 0; -293.434]*10^(-3);     %Control Front

%Propeller arms - rotated
c_1 = TcgCatia*c_1;
c1 = transpose(c_1);
c_2 = TcgCatia*c_2;
c2 = transpose(c_2);
c_3 = TcgCatia*c_3;
c3 = transpose(c_3);

xc_1 = c1(1);
zc_1 = c1(3);

xc_2 = c2(1);
zc_2 = c2(3);

xc_3 = c3(1);
zc_3 = c3(3);

A_control = [1 1 1;
    zc_1 zc_2 zc_3;
    xc_1 xc_2 xc_3];
A_cinv = inv(A_control);
force_control = [F_y; M_x; M_z];
controlvec = A_cinv*force_control;
F_c1 = controlvec(1);
F_c2 = controlvec(2);
F_c3 = controlvec(3);
end

== matlab function Trial_Merge_Unsuccessful/Subsystem11/Subsystem/Resettable Subsystem1/Subsystem1/Subsystem3/MATLAB Function7 ==
  data: F1 input; F_z output; F2 input; M_y output; F3 input
function [F_z, M_y] = fcn(F1, F2, F3)
xt_1 = 1.2598;
xb_1 = 2.2598;
xt_3 = -1.3402;
x_t1 = xt_1;
x_b1 = xb_1;
x_t3 = xt_3;

M_y = -100;
F_z = 0;

A_mat = [1 1;
    xt_1 xb_1];

A_inv = inv(A_mat);

force = [F1; F2];

back = A_mat*force;
backtrack = [4*F3; 4*F3*xt_3];
forceback = back+backtrack;
F_z = forceback(1);
M_y = forceback(2) + 0.15;
end

== matlab function Trial_Merge_Unsuccessful/Subsystem11/Subsystem/Resettable Subsystem1/Subsystem1/Subsystem3/MATLAB Function8 ==
  data: F_c1 input; F_y output; M_x output; F_c2 input; F_c3 input; M_z output
function [F_y, M_x, M_z] = fcn(F_c1, F_c2, F_c3)

%CATIA trans
TcgCatia = [1 0 0;
    0 -1 0;
    0 0 -1];

%Propeller arms - changed due to CATIA errors
c_1 = [-640.1998; 0; 506.566]*10^(-3);      %Control Back Top
c_2 = [-1040.1998; 0; -493.434]*10^(-3);    %Control Back Bottom
c_3 = [2259.8002; 0; -293.434]*10^(-3);     %Control Front

%Propeller arms - rotated
c_1 = TcgCatia*c_1;
c1 = transpose(c_1);
c_2 = TcgCatia*c_2;
c2 = transpose(c_2);
c_3 = TcgCatia*c_3;
c3 = transpose(c_3);

xc_1 = c1(1);
zc_1 = c1(3);

xc_2 = c2(1);
zc_2 = c2(3);

xc_3 = c3(1);
zc_3 = c3(3);


Control_forces = [F_c1; F_c2; F_c3];

A_control = [1 1 1;
        zc_1 zc_2 zc_3;
        xc_1 xc_2 xc_3]; 
Control_vec_2 = A_control*Control_forces;
F_y = Control_vec_2(1);
M_x = Control_vec_2(2);
M_z = Control_vec_2(3);
end

== matlab function Trial_Merge_Unsuccessful/Subsystem11/Subsystem/Resettable Subsystem1/Subsystem1/Subsystem3/MATLAB Function9 ==
  data: Ft1 input; F1 output; Ft2 input; F2 output; F3 output; Ft3 input; Ft4 input; Fb1 input; Fb2 input; Fb3 input; Fb4 input
function [F1, F2, F3] = fcn(Ft1, Ft2, Ft3, Ft4, Fb1, Fb2, Fb3, Fb4)
%F3 is one prop
%F1 is two props
%F2 is two props
F1 = 2*Ft1;
F2 = 2*Fb1;
F3 = Ft3;
end

== matlab function Trial_Merge_Unsuccessful/Subsystem11/Subsystem/Resettable Subsystem1/Subsystem3/MATLAB Function10 ==
  settings: updateMethod=DISCRETE
  data: xvel input; yvel input; zvel input; wx output; accx input; accy input; accz input; wy output; wz output
function [wx, wy, wz]  = fungyroscope(xvel, yvel, zvel, accx, accy, accz)
   
    % Create gyroscope sensor object
    params = gyroparams;         
    
    % Parameters for simulated signal
    N = 1;       % Number of samples
    Fs = 100;       % Sampling rate
    Fc = 0.25;      % Sinusoidal frequency
    
    % Create arrays
    t = (0:(1/Fs):((N-1)/Fs)).';
    acc = [accx, accy, accz];          % Input accelerations
    angvel = [xvel,yvel,zvel];
    %angvel(:,1) = 8*sin(2*pi*Fc*t);
    
    % Generate gyroscopic data
    imu = imuSensor('SampleRate', Fs, 'Gyroscope', params);
    %imu.Gyroscope.MeasurementRange = 1000;   % Maximum angular velocity gyroscope can measure
    %imu.Gyroscope.Resolution = 1/Fs;           % Step size of digital measurements
    
    % Biases
    
    %imu.Gyroscope.BiasInstability = 0.012 * 3.14159 / 180;       % rad/hr
    %imu.Gyroscope.NoiseDensity = 0.15 * 3.14159 / 180;          % rad/s
    %imu.Gyroscope.RandomWalk = 0.017 * 3.14159 / 180;           % rad/sqrt(hr)
    %imu.Gyroscope.TemperatureBias = 0.25 * 3.14159 / 180;       % rad/s
    %imu.Gyroscope.AccelerationBias = 0.3;
    
    % Define real accelerations
    %acc(:,1) = 1;
    [~, gyroData] = imu(acc, angvel, eye(3));
    
    wx = gyroData(1);
    wy = gyroData(2);
    wz = gyroData(3);

end

== matlab function Trial_Merge_Unsuccessful/Subsystem11/Subsystem/Resettable Subsystem1/Subsystem4/MATLAB Function2 ==
  data: theta_x input; Transformation_Mat output; theta_y input; theta_z input
function Transformation_Mat  = Euler(theta_x, theta_y, theta_z)

a = cos(theta_x)*cos(theta_z);
b = cos(theta_x)*sin(theta_z);
c = - sin(theta_x);
d = sin(theta_y)*sin(theta_x)*cos(theta_z) - cos(theta_y)*sin(theta_z);
e = sin(theta_y)*sin(theta_x)*sin(theta_z) + cos(theta_y)*cos(theta_z);
f = sin(theta_y)*cos(theta_x);
g = cos(theta_y)*sin(theta_x)*cos(theta_z) + sin(theta_y)*sin(theta_z);
h = cos(theta_y)*sin(theta_x)*sin(theta_z) - sin(theta_y)*cos(theta_z);
i = cos(theta_y)*cos(theta_x);

Transformation_Mat = [a b c;
    d e f;
    g h i];


end

== matlab function Trial_Merge_Unsuccessful/Subsystem11/Subsystem/Resettable Subsystem1/Subsystem4/MATLAB Function3 ==
  data: theta_x input; Transformation_Mat output; theta_y input; theta_z input
function Transformation_Mat  = Euler(theta_x, theta_y, theta_z)

a = cos(theta_x)*cos(theta_z);
b = cos(theta_x)*sin(theta_z);
c = - sin(theta_x);
d = sin(theta_y)*sin(theta_x)*cos(theta_z) - cos(theta_y)*sin(theta_z);
e = sin(theta_y)*sin(theta_x)*sin(theta_z) + cos(theta_y)*cos(theta_z);
f = sin(theta_y)*cos(theta_x);
g = cos(theta_y)*sin(theta_x)*cos(theta_z) + sin(theta_y)*sin(theta_z);
h = cos(theta_y)*sin(theta_x)*sin(theta_z) - sin(theta_y)*cos(theta_z);
i = cos(theta_y)*cos(theta_x);

Transformation_Mat = [a b c;
    d e f;
    g h i];


end

== matlab function Trial_Merge_Unsuccessful/Subsystem11/Subsystem/Resettable Subsystem/Subsystem/MATLAB Function5 ==
  data: M_y input; F1 output; F_z input; F2 output; F3 output
function [F1, F2, F3] = fcn(M_y, F_z)
xt_1 = 1.2598;
xb_1 = 2.2598;
xt_3 = -1.3402;
x_t1 = xt_1;
x_b1 = xb_1;
x_t3 = xt_3;



A_mat = [1 1;
    xt_1 xb_1];

A_inv = inv(A_mat);

p_0 = 0.2;
p_minus1 = 0;
step = 1000;
Converged = 0;
p_list = [];
x_list = [];
y_list = [];
J_list = [];
Fzz =[];
Myy =[];
while Converged == 0
    B = [(F_z - 4*p_0); (M_y - 4*p_0*xt_3)];
    force_0 = (A_inv*B);
    J_0 = sqrt(force_0(1)^2 + force_0(2)^2 + p_0^2);
    back = A_mat*force_0;
    backtrack = [4*p_0; 4*p_0*xt_3];
    forceback = back+backtrack;
    diff = sum(abs(forceback - [F_z; M_y]));
    if diff > 10^(-7)
        disp('Error')
        break
    end
    force = force_0;
    J = J_0;
    p = p_0;
    
    p_1 = p_0 + step;
    B = [(F_z - 4*p_1); (M_y - 4*p_1*xt_3)];
    force_1 = (A_inv*B);
    J_1 = sqrt(force_1(1)^2 + force_1(2)^2 + p_1^2);
    back = A_mat*force_1;
    backtrack = [4*p_1; 4*p_1*xt_3];
    forceback = back+backtrack;
    diff = sum(abs(forceback - [F_z; M_y]));
    if diff > 10^(-7)
        disp('Error')
        break
    end
    if J_1 < J_0
        force = force_1;
        J = J_1;
        p = p_1;
    end
    
    p_2 = p_0 - step;
    B = [(F_z - 4*p_2); (M_y - 4*p_2*xt_3)];
    force_2 = (A_inv*B);
    J_2 = sqrt(force_2(1)^2 + force_2(2)^2 + p_2^2);
    back = A_mat*force_2;
    backtrack = [4*p_2; 4*p_2*xt_3];
    forceback = back+backtrack;
    diff = sum(abs(forceback - [F_z; M_y]));
    if diff > 10^(-7)
        disp('Error')
        break
    end
    if J_2 < J_0 && J_2 < J_1
        force = force_2;
        J = J_2;
        p = p_2;
    end
    
    if p_minus1 < p_0 && p_0 < p
        step = step;
    elseif p_minus1 > p_0 && p_0 > p
        step = step;
    else
        step = step*0.9;
    end
        
    p_minus1 = p_0;
    p_0 = p;
    p_list = [p_list; p_0];
    x_list = [x_list; force(1)];
    y_list = [y_list; force(2)];
    J_list = [J_list; J];
    if step < abs(min([F_z,M_y])*10^(-9))
        Converged = 1;
    end
    
    
end

F1 = x_list(length(x_list));
F2 = y_list(length(y_list));
F3 = p_0;
end

== matlab function Trial_Merge_Unsuccessful/Subsystem11/Subsystem/Resettable Subsystem/Subsystem/Subsystem/MATLAB Function ==
  data: My input; Ft1 output; Fz input; Ft2 output; Ft3 output; Ft4 output; Fb1 output; Fb2 output; Fb3 output; Fb4 output
function [Ft1, Ft2, Ft3, Ft4, Fb1, Fb2, Fb3, Fb4] = fixingpropulsionsmess(My, Fz)
xt_1 = 1.2598;
xb_1 = 2.2598;
xt_3 = -1.3402;
xb_3 = -1.3402;
x_t1 = xt_1;
x_b1 = xb_1;
x_t3 = xt_3;
x_b3 = xb_3;;

%alpha_1 = (-2*xt_1*(1/((xt_1/xb_1)-1))*(2 - (2*xb_3/xb_1)) - 4*xb_3)^2;
%alpha_2 = ((1/((xt_1/xb_1)-1))*(2-(2*xb_3/xb_1)))^2;
%alpha = alpha_1 + alpha_2;

%beta_1 = 2*My*((1/(2*xb_1))*(1 - (xt_1/xb_1)*(1/((xt_1/xb_1) -1))));
%beta_2 = 2*My*(1/((xt_1/xb_1) -1))*(1/(2*xb_1))*(1/((xt_1/xb_1) -1))*(2 - ((2*xb_3)/x_b1));
%beta_3 = 2*Fz*(1/(2*xb_1)*xt_1*(1/(xt_1/xb_1 -1)));
%beta_4 = 2*Fz*(-1/2*(1/(xt_1/xb_1 -1))*(1/(xt_1/xb_1 -1))*(2-2*xb_3/xb_1));
%beta = beta_1 + beta_2 + beta_3 + beta_4;

%a = beta/(2*alpha);
%y = 1/(2*xb_1)*(My - 2*xt_1*(1/(xt_1/xb_1 -1))*(-0.5*Fz + 2*(2 - 2*xb_3/xb_1)*a + 1/(2*xb_1)*My) - 4*xb_3*a);
%x = (1/(xt_1/xb_1 -1))*(-0.5*Fz + (2 - 2*xb_3/xb_1)*a + 1/(2*xb_1)*My);

a_num = 2/((2*xb_1 - 2*xt_1)^2) *(2*(4*xt_1 - 4*xb_3)*(My - Fz*0.5)) + 2*Fz + (4*My - Fz*(2 + 4*xt_1 - 4*xb_3))/(2*xb_1 - 2*xt_1);
a_den = -(2/((2*xb_1 - 2*xt_1)^2)*2*((4*xt_1 - 4*xb_3)^2) + 10 + (8*(4*xt_1 - 4*xb_3))/(-2*xt_1 + 2*xb_1));
a = a_num/a_den;

y = 1/(-2*xt_1 + 2*xb_1)*(a*(4*xt_1 - 4*xb_3) + My - 0.5*Fz);
x = -y - 2*a + Fz/2;
z = a;

Ft1 = x;
Ft2 = Ft1;
Ft3 = a;
Ft4 = Ft3;
Fb1 = y;
Fb2 = Fb1;
Fb3 = Ft3;
Fb4 = Ft3;
end

== matlab function Trial_Merge_Unsuccessful/Subsystem5/Subsystem/MATLAB Function ==
  data: My input; Ft1 output; Fz input; Ft2 output; Ft3 output; Ft4 output; Fb1 output; Fb2 output; Fb3 output; Fb4 output
function [Ft1, Ft2, Ft3, Ft4, Fb1, Fb2, Fb3, Fb4] = fixingpropulsionsmess(My, Fz)
xt_1 = 1.2598;
xb_1 = 2.2598;
xt_3 = -1.3402;
xb_3 = -1.3402;
x_t1 = xt_1;
x_b1 = xb_1;
x_t3 = xt_3;
x_b3 = xb_3;;

%alpha_1 = (-2*xt_1*(1/((xt_1/xb_1)-1))*(2 - (2*xb_3/xb_1)) - 4*xb_3)^2;
%alpha_2 = ((1/((xt_1/xb_1)-1))*(2-(2*xb_3/xb_1)))^2;
%alpha = alpha_1 + alpha_2;

%beta_1 = 2*My*((1/(2*xb_1))*(1 - (xt_1/xb_1)*(1/((xt_1/xb_1) -1))));
%beta_2 = 2*My*(1/((xt_1/xb_1) -1))*(1/(2*xb_1))*(1/((xt_1/xb_1) -1))*(2 - ((2*xb_3)/x_b1));
%beta_3 = 2*Fz*(1/(2*xb_1)*xt_1*(1/(xt_1/xb_1 -1)));
%beta_4 = 2*Fz*(-1/2*(1/(xt_1/xb_1 -1))*(1/(xt_1/xb_1 -1))*(2-2*xb_3/xb_1));
%beta = beta_1 + beta_2 + beta_3 + beta_4;

%a = beta/(2*alpha);
%y = 1/(2*xb_1)*(My - 2*xt_1*(1/(xt_1/xb_1 -1))*(-0.5*Fz + 2*(2 - 2*xb_3/xb_1)*a + 1/(2*xb_1)*My) - 4*xb_3*a);
%x = (1/(xt_1/xb_1 -1))*(-0.5*Fz + (2 - 2*xb_3/xb_1)*a + 1/(2*xb_1)*My);

a_num = 2/((2*xb_1 - 2*xt_1)^2) *(2*(4*xt_1 - 4*xb_3)*(My - Fz*0.5)) + 2*Fz + (4*My - Fz*(2 + 4*xt_1 - 4*xb_3))/(2*xb_1 - 2*xt_1);
a_den = -(2/((2*xb_1 - 2*xt_1)^2)*2*((4*xt_1 - 4*xb_3)^2) + 10 + (8*(4*xt_1 - 4*xb_3))/(-2*xt_1 + 2*xb_1));
a = a_num/a_den;

y = 1/(-2*xt_1 + 2*xb_1)*(a*(4*xt_1 - 4*xb_3) + My - 0.5*Fz);
x = -y - 2*a + Fz/2;
z = a;

Ft1 = x;
Ft2 = Ft1;
Ft3 = a;
Ft4 = Ft3;
Fb1 = y;
Fb2 = Fb1;
Fb3 = Ft3;
Fb4 = Ft3;
end

== matlab function Trial_Merge_Unsuccessful/Subsystem11/Subsystem/Resettable Subsystem/Subsystem/Subsystem/MATLAB Function6 ==
  data: F_y input; F_c1 output; M_x input; M_z input; F_c2 output; F_c3 output
function [F_c1, F_c2, F_c3] = fcn(F_y, M_x, M_z)
%CATIA trans
TcgCatia = [1 0 0;
    0 -1 0;
    0 0 -1];

%Propeller arms - changed due to CATIA errors
c_1 = [-640.1998; 0; 506.566]*10^(-3);      %Control Back Top
c_2 = [-1040.1998; 0; -493.434]*10^(-3);    %Control Back Bottom
c_3 = [2259.8002; 0; -293.434]*10^(-3);     %Control Front

%Propeller arms - rotated
c_1 = TcgCatia*c_1;
c1 = transpose(c_1);
c_2 = TcgCatia*c_2;
c2 = transpose(c_2);
c_3 = TcgCatia*c_3;
c3 = transpose(c_3);

xc_1 = c1(1);
zc_1 = c1(3);

xc_2 = c2(1);
zc_2 = c2(3);

xc_3 = c3(1);
zc_3 = c3(3);

A_control = [1 1 1;
    zc_1 zc_2 zc_3;
    xc_1 xc_2 xc_3];
A_cinv = inv(A_control);
force_control = [F_y; M_x; M_z];
controlvec = A_cinv*force_control;
F_c1 = controlvec(1);
F_c2 = controlvec(2);
F_c3 = controlvec(3);
end

== matlab function Trial_Merge_Unsuccessful/Subsystem11/Subsystem/Resettable Subsystem/Subsystem/Subsystem3/MATLAB Function7 ==
  data: F1 input; F_z output; F2 input; M_y output; F3 input
function [F_z, M_y] = fcn(F1, F2, F3)
xt_1 = 1.2598;
xb_1 = 2.2598;
xt_3 = -1.3402;
x_t1 = xt_1;
x_b1 = xb_1;
x_t3 = xt_3;

M_y = -100;
F_z = 0;

A_mat = [1 1;
    xt_1 xb_1];

A_inv = inv(A_mat);

force = [F1; F2];

back = A_mat*force;
backtrack = [4*F3; 4*F3*xt_3];
forceback = back+backtrack;
F_z = forceback(1);
M_y = forceback(2) + 0.15;
end

== matlab function Trial_Merge_Unsuccessful/Subsystem11/Subsystem/Resettable Subsystem/Subsystem/Subsystem3/MATLAB Function8 ==
  data: F_c1 input; F_y output; M_x output; F_c2 input; F_c3 input; M_z output
function [F_y, M_x, M_z] = fcn(F_c1, F_c2, F_c3)

%CATIA trans
TcgCatia = [1 0 0;
    0 -1 0;
    0 0 -1];

%Propeller arms - changed due to CATIA errors
c_1 = [-640.1998; 0; 506.566]*10^(-3);      %Control Back Top
c_2 = [-1040.1998; 0; -493.434]*10^(-3);    %Control Back Bottom
c_3 = [2259.8002; 0; -293.434]*10^(-3);     %Control Front

%Propeller arms - rotated
c_1 = TcgCatia*c_1;
c1 = transpose(c_1);
c_2 = TcgCatia*c_2;
c2 = transpose(c_2);
c_3 = TcgCatia*c_3;
c3 = transpose(c_3);

xc_1 = c1(1);
zc_1 = c1(3);

xc_2 = c2(1);
zc_2 = c2(3);

xc_3 = c3(1);
zc_3 = c3(3);


Control_forces = [F_c1; F_c2; F_c3];

A_control = [1 1 1;
        zc_1 zc_2 zc_3;
        xc_1 xc_2 xc_3]; 
Control_vec_2 = A_control*Control_forces;
F_y = Control_vec_2(1);
M_x = Control_vec_2(2);
M_z = Control_vec_2(3);
end
